simulink model "airbus300"  (R2024a)
settings: Solver=VariableStepAuto  StartTime=0.0  StopTime=10.0  RelTol=1e-3
settings Model: Creator=cunis  LastModifiedBy=cunis

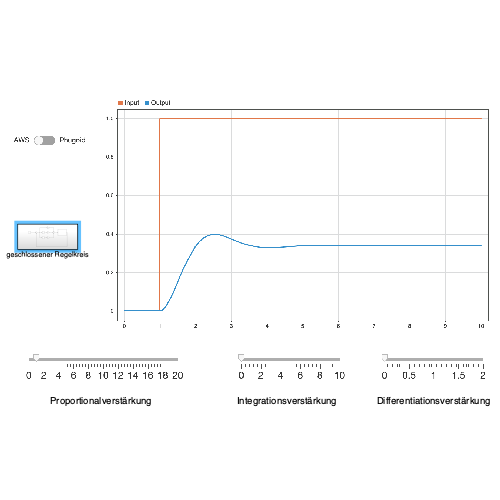
[thumbnail: Simulink's stored preview of the top-level diagram]
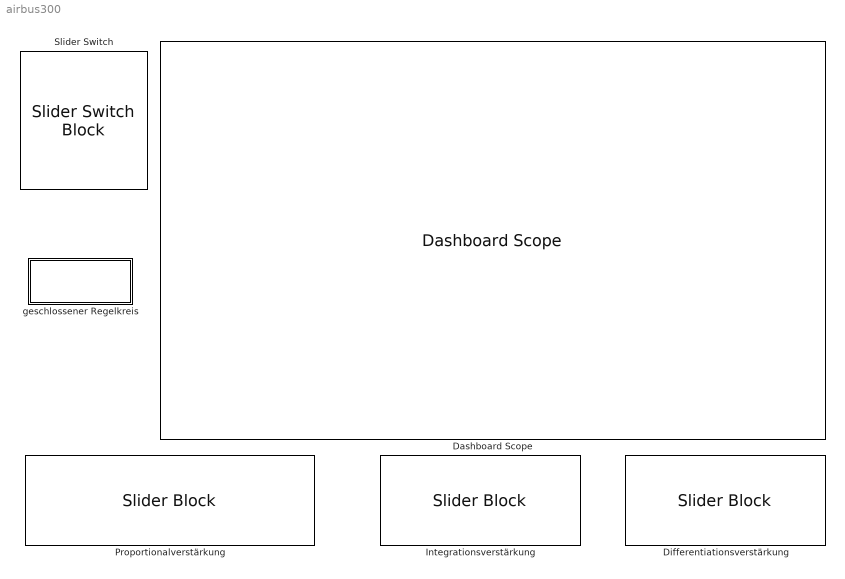
== system airbus300 ==
  Dashboard Scope : DashboardScope
  Differentiationsverstärkung : SliderBlock  LabelPosition=Hide  ScaleMax=2  TickInterval=0.5
  Integrationsverstärkung : SliderBlock  LabelPosition=Hide  ScaleMax=10
  Proportionalverstärkung : SliderBlock  LabelPosition=Hide  ScaleMax=20
  Slider Switch : SliderSwitchBlock  LabelPosition=Hide
      settings: Values={{'AWS', 'Phugoid'}, [1 -1]}
  geschlossener Regelkreis : Subsystem

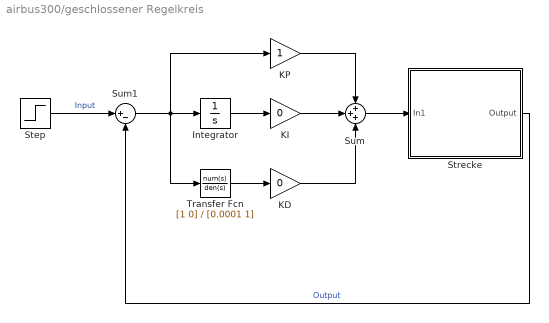
== system airbus300/geschlossener Regelkreis ==
  Integrator : Integrator
  KD : Gain  Gain=0
  KI : Gain  Gain=0
  KP : Gain
  Step : Step  SampleTime=0
  Strecke : Subsystem
  Sum : Sum  Inputs=+++
  Sum1 : Sum  Inputs=|+-
  Transfer Fcn : TransferFcn  Numerator=[1 0]  Denominator=[0.0001 1]
  wires:
  KP/1 -> Sum/1
  Sum1/1 -> Transfer Fcn/1, Integrator/1, KP/1
  KI/1 -> Sum/2
  Integrator/1 -> KI/1
  Transfer Fcn/1 -> KD/1
  KD/1 -> Sum/3
  Step/1 -> Sum1/1  "Input"
  Sum/1 -> Strecke/1(In1)
  Strecke/1(Output) -> Sum1/2  "Output"

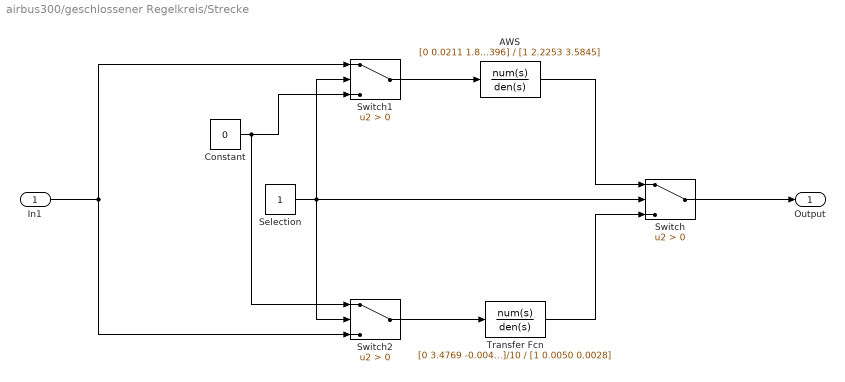
== system airbus300/geschlossener Regelkreis/Strecke ==
  In1 : Inport
  AWS : TransferFcn  Numerator=[0 0.0211 1.8396]  Denominator=[1 2.2253 3.5845]
  Constant : Constant  Value=0
  Selection : Constant
  Switch : Switch  Criteria=u2 > Threshold  SaturateOnIntegerOverflow=off  InputSameDT=off
  Switch1 : Switch  Criteria=u2 > Threshold  SaturateOnIntegerOverflow=off  InputSameDT=off
  Switch2 : Switch  Criteria=u2 > Threshold  SaturateOnIntegerOverflow=off  InputSameDT=off
  Transfer Fcn : TransferFcn  Numerator=[0 3.4769 -0.0049]/10  Denominator=[1 0.0050 0.0028]
  Output : Outport
  wires:
  Switch/1 -> Output/1
  In1/1 -> Switch2/3, Switch1/1
  Selection/1 -> Switch2/2, Switch/2, Switch1/2
  AWS/1 -> Switch/1
  Transfer Fcn/1 -> Switch/3
  Switch1/1 -> AWS/1
  Switch2/1 -> Transfer Fcn/1
  Constant/1 -> Switch2/1, Switch1/3
